simulink model "csma_stateflow"  (R2021a)
settings: Solver=VariableStepAuto  StartTime=0.0  StopTime=10.0  RelTol=1e-3
settings Model: EnablePacing=on  OrderedModelArguments=off  Creator=411sa  LastModifiedBy=mluser

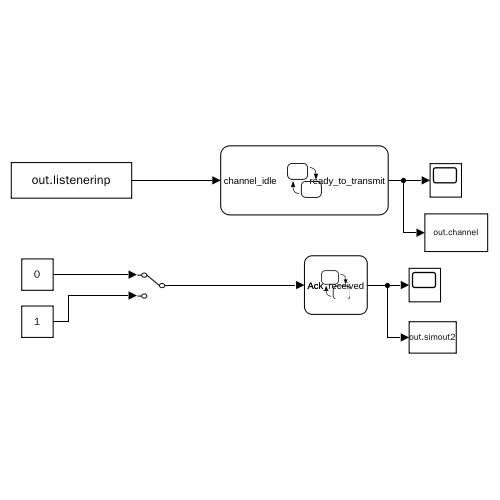
[thumbnail: Simulink's stored preview of the top-level diagram]
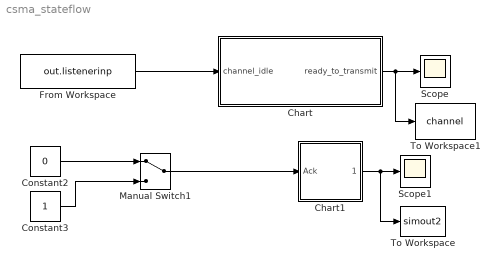
== system csma_stateflow ==
  Chart : Stateflow chart  TreatAsAtomicUnit=on
  Chart1 : Stateflow chart  TreatAsAtomicUnit=on
  Constant2 : Constant  Value=0
  Constant3 : Constant
  From Workspace : FromWorkspace  VariableName=out.listenerinp  OutDataTypeStr=double  Interpolate=off  OutputAfterFinalValue=Holding final value
  Manual Switch1 : ManualSwitch
  Scope : Scope
  Scope1 : Scope
  To Workspace : ToWorkspace  VariableName=simout2  SaveFormat=Structure With Time  SampleTime=-1
  To Workspace1 : ToWorkspace  VariableName=channel  SaveFormat=Structure With Time  SampleTime=-1
  wires:
  Manual Switch1/1 -> Chart1/1(Ack)
  Constant3/1 -> Manual Switch1/2
  Constant2/1 -> Manual Switch1/1
  Chart1/1(Ack_received) -> To Workspace/1, Scope1/1
  From Workspace/1 -> Chart/1(channel_idle)
  Chart/1(ready_to_transmit) -> To Workspace1/1, Scope/1

== stateflow chart csma_stateflow/Chart1 ==
  state maxAckWaitDuration
    maxAckWait=maxAckWait-1;
  state Success
    Ack_received=1
  state Wait_for_unit_time
    unit_time=unit_time-1;
  state Failure
    Ack_received=0
  (default) -> maxAckWaitDuration : {maxAckWait=50}
  maxAckWaitDuration -> Success [order 1] : [Ack==1]
  Wait_for_unit_time -> Success [order 1] : [Ack == 1]
  maxAckWaitDuration -> Wait_for_unit_time [order 2] : [maxAckWait>=0]{unit_time=50}
  Wait_for_unit_time -> Failure [order 3] : [unit_time<=0]
  Wait_for_unit_time -> Wait_for_unit_time [order 2] : [unit_time>0]
  data: Ack input; maxAckWait local; Ack_received output; unit_time local

== stateflow chart csma_stateflow/Chart ==
  state UpdateNBandBE_
    NB=NB+1;
    be=min(be+1,macMinBE);
  state Initialisation_
    NB=0;
    macMinBE = 50;
    be= 5;
    maxBackoffs=10;
  state Random_Delay_
    rand_delay=rand_delay-1;
  state Transmit_
    ready_to_transmit=1;
  state Unit_Time
    unit_time=unit_time-1;
  (default) -> Initialisation_
  UpdateNBandBE_ -> Random_Delay_ : [NB<=maxBackoffs]
      | {rand_delay=randi((2^be)-1)}
  Random_Delay_ -> UpdateNBandBE_ [order 3] : [channel_idle==0]
  Random_Delay_ -> Transmit_ [order 1] : [channel_idle==1 && rand_delay<=0]
  Initialisation_ -> Random_Delay_ : {rand_delay=randi((2^be)-1)}
  Unit_Time -> Random_Delay_ [order 2] : [unit_time<=0]
  Random_Delay_ -> Unit_Time [order 2] : [rand_delay>0]{unit_time=5}
  Unit_Time -> Unit_Time [order 1] : [unit_time>0]
  data: channel_idle input; be local; macMinBE local; maxAckWait local; NB local; BE local; rand_delay local; message1 local; message local; ChartMode local Enum: ChartModeType; maxBackoffs local; ready_to_transmit output; unit_time local
  events: initialisation local FUNCTION_CALL_EVENT; initialisation1 local FUNCTION_CALL_EVENT; event local FUNCTION_CALL_EVENT; event1 local FUNCTION_CALL_EVENT; event2 local FUNCTION_CALL_EVENT
